simulink model "BLDC"  (R2023a)
settings: Solver=VariableStepAuto  StartTime=0.0  StopTime=36  RelTol=1e-3
undefined symbols (not defined in the file): J_rot, K_m, K_w, L_ph, P_amt, R_ph
settings Model: Creator=Artem Sannikov  LastModifiedBy=Artem Sannikov

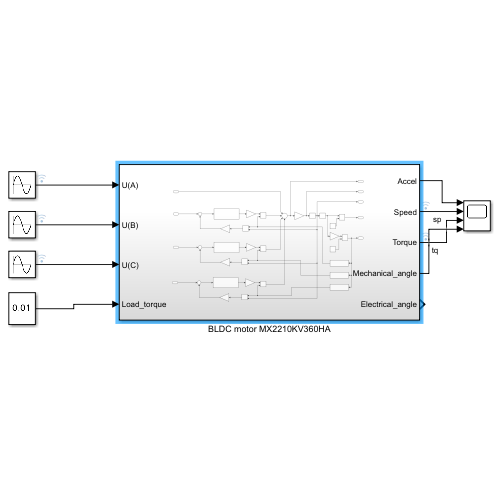
[thumbnail: Simulink's stored preview of the top-level diagram]
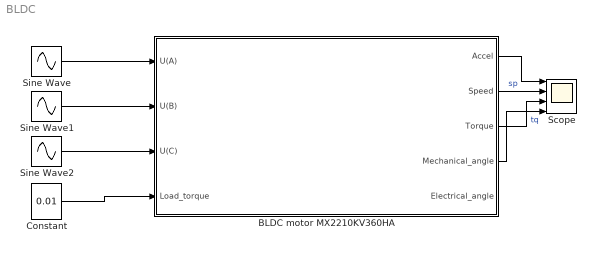
== system BLDC ==
  BLDC motor MX2210KV360HA : Subsystem
  Constant : Constant  Value=0.01
  Scope : Scope  NumInputPorts=4
  Sine Wave : Sin  Amplitude=12  Frequency=50  SampleTime=0
  Sine Wave1 : Sin  Amplitude=12  Frequency=50  Phase=2/3*pi  SampleTime=0
  Sine Wave2 : Sin  Amplitude=12  Frequency=50  Phase=4/3*pi  SampleTime=0
  wires:
  Sine Wave1/1 -> BLDC motor MX2210KV360HA/2(U(B))
  Constant/1 -> BLDC motor MX2210KV360HA/4(Load_torque)
  BLDC motor MX2210KV360HA/2(Speed) -> Scope/2  "sp"
  BLDC motor MX2210KV360HA/3(Torque) -> Scope/3  "tq"
  BLDC motor MX2210KV360HA/1(Accel) -> Scope/1
  Sine Wave2/1 -> BLDC motor MX2210KV360HA/3(U(C))
  Sine Wave/1 -> BLDC motor MX2210KV360HA/1(U(A))
  BLDC motor MX2210KV360HA/4(Mechanical_angle) -> Scope/4

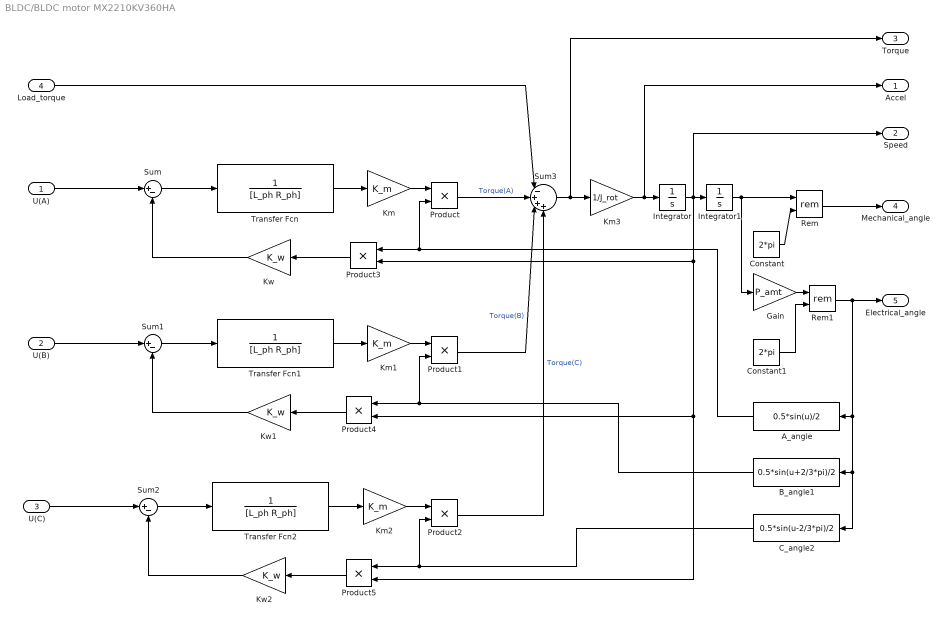
== system BLDC/BLDC motor MX2210KV360HA ==
  U(A) : Inport
  U(B) : Inport  Port=2
  U(C) : Inport  Port=3
  Load_torque : Inport  Port=4
  A_angle : Fcn  Expr=0.5*sin(u)/2
  B_angle1 : Fcn  Expr=0.5*sin(u+2/3*pi)/2
  C_angle2 : Fcn  Expr=0.5*sin(u-2/3*pi)/2
  Constant : Constant  Value=2*pi
  Constant1 : Constant  Value=2*pi
  Gain : Gain  Gain=P_amt
  Integrator : Integrator
  Integrator1 : Integrator
  Km : Gain  Gain=K_m
  Km1 : Gain  Gain=K_m
  Km2 : Gain  Gain=K_m
  Km3 : Gain  Gain=1/J_rot
  Kw : Gain  Gain=K_w
  Kw1 : Gain  Gain=K_w
  Kw2 : Gain  Gain=K_w
  Product{,1..5} (6 alike) : Product
  Rem : Math  Operator=rem
  Rem1 : Math  Operator=rem
  Sum : Sum  Inputs=|+-
  Sum1 : Sum  Inputs=|+-
  Sum2 : Sum  Inputs=|+-
  Sum3 : Sum  Inputs=|-+++
  Transfer Fcn : TransferFcn  Denominator=[L_ph R_ph]
  Transfer Fcn1 : TransferFcn  Denominator=[L_ph R_ph]
  Transfer Fcn2 : TransferFcn  Denominator=[L_ph R_ph]
  Accel : Outport
  Speed : Outport  Port=2
  Torque : Outport  Port=3
  Mechanical_angle : Outport  Port=4
  Electrical_angle : Outport  Port=5
  wires:
  Sum/1 -> Transfer Fcn/1
  U(A)/1 -> Sum/1
  Transfer Fcn/1 -> Km/1
  Kw/1 -> Sum/2
  Transfer Fcn1/1 -> Km1/1
  Sum1/1 -> Transfer Fcn1/1
  U(B)/1 -> Sum1/1
  Kw1/1 -> Sum1/2
  Kw2/1 -> Sum2/2
  Sum2/1 -> Transfer Fcn2/1
  Transfer Fcn2/1 -> Km2/1
  U(C)/1 -> Sum2/1
  Km/1 -> Product/1
  Product/1 -> Sum3/2  "Torque(A)"
  Km1/1 -> Product1/1
  Product1/1 -> Sum3/3  "Torque(B)"
  Km2/1 -> Product2/1
  Product2/1 -> Sum3/4  "Torque(C)"
  Sum3/1 -> Torque/1, Km3/1
  Km3/1 -> Accel/1, Integrator/1
  Load_torque/1 -> Sum3/1
  Product3/1 -> Kw/1
  Integrator/1 -> Product5/2, Product4/2, Product3/2, Speed/1, Integrator1/1
  Integrator1/1 -> Gain/1, Rem/1
  Constant/1 -> Rem/2
  Rem/1 -> Mechanical_angle/1
  Gain/1 -> Rem1/1
  Rem1/1 -> C_angle2/1, B_angle1/1, A_angle/1, Electrical_angle/1
  Constant1/1 -> Rem1/2
  Product4/1 -> Kw1/1
  Product5/1 -> Kw2/1
  A_angle/1 -> Product/2, Product3/1
  B_angle1/1 -> Product1/2, Product4/1
  C_angle2/1 -> Product2/2, Product5/1
